simulink model "SMC_Plant"  (R2021a)
settings: Solver=ode45  StartTime=0.0  StopTime=300  MaxStep=0.2  RelTol=1e-5
settings Model: Creator=Denilson Nicolau  LastModifiedBy=Denilson Nicolau

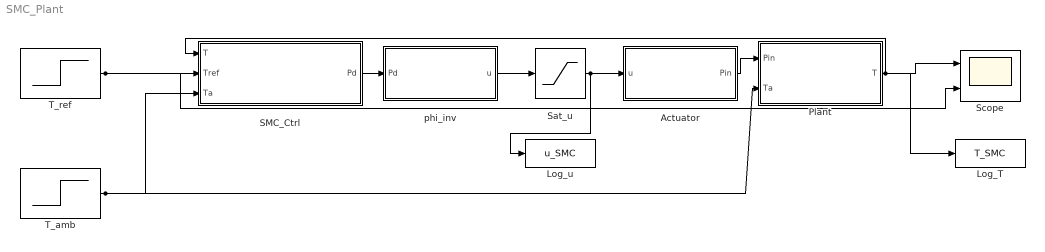
== system SMC_Plant ==
  Actuator : MATLAB Function  TreatAsAtomicUnit=on
  Log_T : ToWorkspace  VariableName=T_SMC  SaveFormat=Timeseries  SampleTime=-1
  Log_u : ToWorkspace  VariableName=u_SMC  SaveFormat=Timeseries  SampleTime=-1
  Plant : Subsystem
  SMC_Ctrl : Subsystem
  Sat_u : Saturate  UpperLimit=1.057  LowerLimit=0
  Scope : Scope  NumInputPorts=2
  T_amb : Step  Time=150  Before=25  After=30  SampleTime=0
  T_ref : Step  Time=0  Before=25  After=70  SampleTime=0
  phi_inv : MATLAB Function  TreatAsAtomicUnit=on
  wires:
  Plant/1(T) -> SMC_Ctrl/1(T), Scope/1, Log_T/1
  T_ref/1 -> SMC_Ctrl/2(Tref), Scope/2
  T_amb/1 -> SMC_Ctrl/3(Ta), Plant/2(Ta)
  SMC_Ctrl/1(Pd) -> phi_inv/1(Pd)
  phi_inv/1(u) -> Sat_u/1
  Sat_u/1 -> Actuator/1(u), Log_u/1
  Actuator/1(Pin) -> Plant/1(Pin)

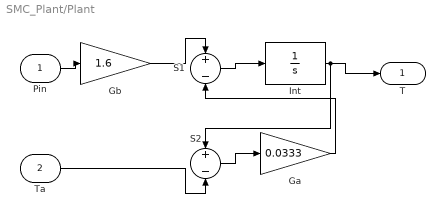
== system SMC_Plant/Plant ==
  Pin : Inport
  Ta : Inport  Port=2
  Ga : Gain  Gain=0.0333
  Gb : Gain  Gain=1.6
  Int : Integrator  InitialCondition=25
  S1 : Sum  Inputs=+-
  S2 : Sum  Inputs=+-
  T : Outport
  wires:
  Pin/1 -> Gb/1
  Gb/1 -> S1/1
  Ga/1 -> S1/2
  S1/1 -> Int/1
  Int/1 -> T/1, S2/1
  Ta/1 -> S2/2
  S2/1 -> Ga/1

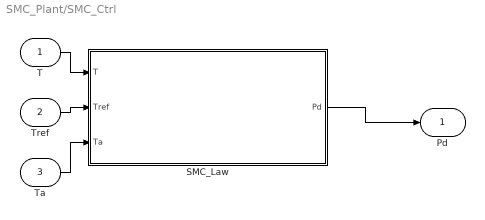
== system SMC_Plant/SMC_Ctrl ==
  T : Inport
  Tref : Inport  Port=2
  Ta : Inport  Port=3
  SMC_Law : MATLAB Function  TreatAsAtomicUnit=on
  Pd : Outport
  wires:
  T/1 -> SMC_Law/1(T)
  Tref/1 -> SMC_Law/2(Tref)
  Ta/1 -> SMC_Law/3(Ta)
  SMC_Law/1(Pd) -> Pd/1

== matlab function SMC_Plant/phi_inv ==
  data: Pd input; u output
function u = phi_inv(Pd)
%%#codegen
  Pd = max(1e-6, min(2.42, double(Pd)));
  u  = (log10(200*Pd) + 1) / 4;
end

== matlab function SMC_Plant/SMC_Ctrl/SMC_Law ==
  data: T input; Pd output; Tref input; Ta input
function Pd = SMC_Law(T, Tref, Ta)
%#codegen
  alpha_hat = 0.0333;
  beta      = 1.6;
  k_s       = 0.7;
  phi_BL    = 0.5;
  s = double(T) - double(Tref);
  if abs(s) > phi_BL
    sat_val = sign(s);
  else
    sat_val = s / phi_BL;
  end
  Pd = (1/beta)*(alpha_hat*(double(T)-double(Ta))-k_s*sat_val);
  Pd = max(0, min(2.42, Pd));
end

== matlab function SMC_Plant/Actuator ==
  data: u input; Pin output
function Pin = Actuator(u)
%%#codegen
  Pin = (10^(4*double(u) - 1)) / 200;
end
